simulink model "basic"  (R2015a)
settings: Solver=ode45  StartTime=0.0  StopTime=10.0  RelTol=1e-3
values from neighbouring files (symbols this model uses):
  D1 = [0 0 0 0 0;0 0 0 0 0]'    [LabCEE.m]
  K = lqr(A, B, Qr, Rr)    [LabCEE.m]    (also in fp_ini.m)
  x_0 = [0.1 0 0 0 0]'    [LabCEE.m]
undefined symbols (not defined in the file or in its folder): A, B, C1
settings Model: Creator=Alunos  LastModifiedBy=Alunos

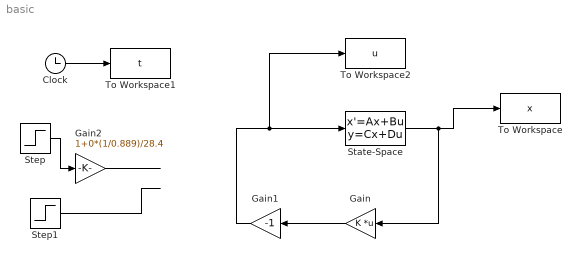
== system basic ==
  Clock : Clock
  Gain : Gain  Gain=K  Multiplication=Matrix(K*u)
  Gain1 : Gain  Gain=-1
  Gain2 : Gain  Gain=1+0*(1/0.889)/28.4
  State-Space : StateSpace  A=A  B=B  C=C1  D=D1  X0=x_0
  Step : Step  Time=20  After=10*(pi/180)*0  SampleTime=0
  Step1 : Step  Time=6  After=0  SampleTime=0
  To Workspace : ToWorkspace  VariableName=x  SampleTime=-1
  To Workspace1 : ToWorkspace  VariableName=t  SampleTime=-1
  To Workspace2 : ToWorkspace  VariableName=u  SampleTime=-1
  wires:
  Clock/1 -> To Workspace1/1
  State-Space/1 -> Gain/1, To Workspace/1
  Gain/1 -> Gain1/1
  Gain1/1 -> To Workspace2/1, State-Space/1
  Step/1 -> Gain2/1
  Gain2/1 -> ?
  Step1/1 -> ?
